simulink model "RateAdaptive_VOOmode"  (R2017b)
settings: Solver=FixedStepAuto  StartTime=0.0  StopTime=inf  FixedStep=0.001  RelTol=1e-3  EnableMultiTasking=on
undefined symbols (not defined in the file): D10, D11, D12, D2, D5, D8, D9, PTA0, PTA2, PTB9, PTC4, PTD0, PTD2, PTD3
libraries: frdmk64flib x10
settings Model: ExtModeTrigDuration=5  Creator=montema2  LastModifiedBy=puerstee
settings OptimizationCC: PassReuseOutputArgsAs=Individual arguments  MaxStackSize=64
settings DebuggingCC: ParameterTunabilityLossMsg=error
settings HardwareCC: ProdBitPerPointer=32  ProdBitPerSizeT=32  ProdBitPerPtrDiffT=32  ProdLargestAtomicInteger=Long  ProdLargestAtomicFloat=Double  ProdWordSize=32  ProdHWDeviceType=ARM Compatible->ARM Cortex
settings SFSimCC: MATLABDynamicMemAlloc=off
settings RTWCC: SystemTargetFile=ert.tlc  HardwareBoard=NXP FRDM-K64F  TemplateMakefile=ert_default_tmf  GenerateReport=on  Toolchain=GNU Tools for ARM Embedded Processors  IncludeHyperlinkInReport=on  LaunchReport=on  GenerateTraceInfo=on  GenerateTraceReport=on  GenerateTraceReportSl=on  GenerateTraceReportSf=on  GenerateTraceReportEml=on
settings CodeAppCC: ForceParamTrailComments=on  IgnoreCustomStorageClasses=off  OperatorAnnotations=on  SimulinkDataObjDesc=on  SFDataObjDesc=on  InsertBlockDesc=on
settings ERTTargetCC: SupportContinuousTime=on

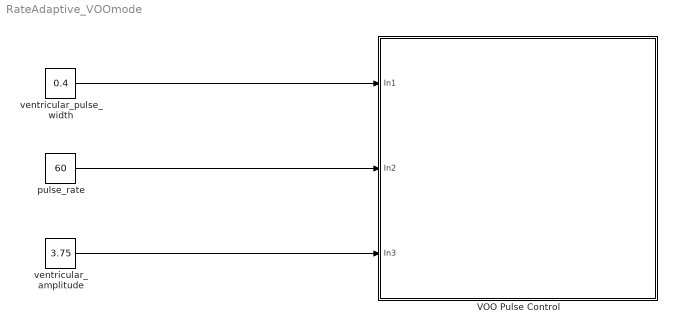
== system RateAdaptive_VOOmode ==
  VOO Pulse Control : Subsystem
  pulse_rate : Constant  Value=60  OutDataTypeStr=single
  ventricular_amplitude : Constant  Value=3.75
  ventricular_pulse_width : Constant  Value=0.4
  wires:
  ventricular_pulse_width/1 -> VOO Pulse Control/1(In1)
  pulse_rate/1 -> VOO Pulse Control/2(In2)
  ventricular_amplitude/1 -> VOO Pulse Control/3(In3)

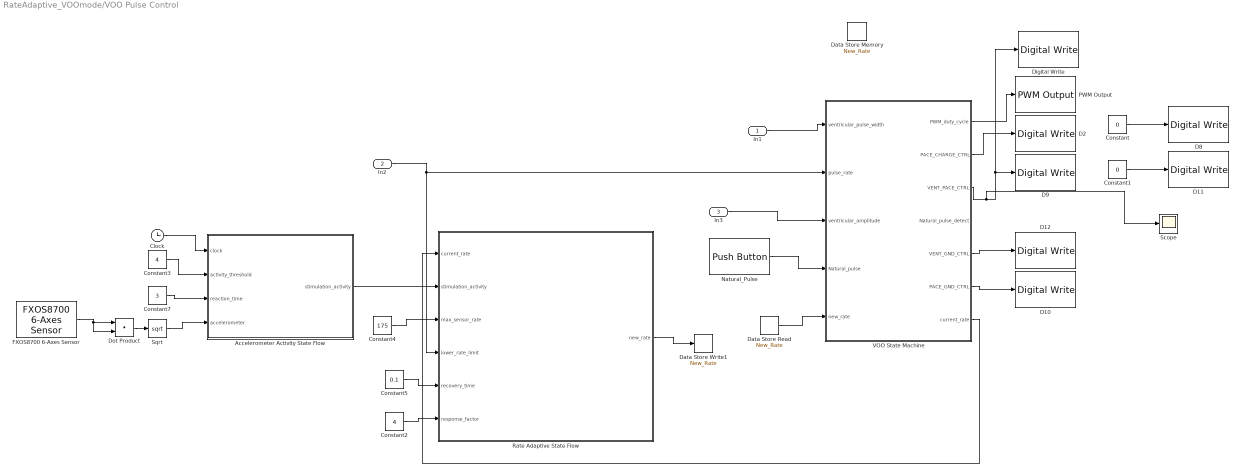
== system RateAdaptive_VOOmode/VOO Pulse Control ==
  In1 : Inport
  In2 : Inport  Port=2
  In3 : Inport  Port=3
  "Accelerometer Activity State Flow " : Stateflow chart  TreatAsAtomicUnit=on
  Clock : Clock
  Constant : Constant  Value=0
  Constant1 : Constant  Value=0
  Constant2 : Constant  Value=4  OutDataTypeStr=single
  Constant3 : Constant  Value=4  OutDataTypeStr=single
  Constant4 : Constant  Value=175  OutDataTypeStr=single
  Constant5 : Constant  Value=0.1  OutDataTypeStr=single
  Constant7 : Constant  Value=3  OutDataTypeStr=single
  D10 : frdmk64flib/Digital Write  Whichpin=PTD0 (D10)
      settings: SourceProductName=Simulink Coder Support Package for NXP FRDM-K64F Board
  D11 : frdmk64flib/Digital Write  Whichpin=PTD2 (D11)
      settings: SourceProductName=Simulink Coder Support Package for NXP FRDM-K64F Board
  D12 : frdmk64flib/Digital Write  Whichpin=PTD3 (D12)
      settings: SourceProductName=Simulink Coder Support Package for NXP FRDM-K64F Board
  D2 : frdmk64flib/Digital Write  Whichpin=PTB9 (D2)
      settings: SourceProductName=Simulink Coder Support Package for NXP FRDM-K64F Board
  D8 : frdmk64flib/Digital Write  Whichpin=PTA0 (D8)
      settings: SourceProductName=Simulink Coder Support Package for NXP FRDM-K64F Board
  D9 : frdmk64flib/Digital Write  Whichpin=PTC4 (D9)
      settings: SourceProductName=Simulink Coder Support Package for NXP FRDM-K64F Board
  Data Store Memory : DataStoreMemory  DataStoreName=New_Rate  ReadBeforeWriteMsg=warning  WriteAfterWriteMsg=warning  WriteAfterReadMsg=warning  InitialValue=60  ShowAdditionalParam=off  OutDataTypeStr=single
  Data Store Read : DataStoreRead  DataStoreName=New_Rate  DataStoreElements=New_Rate
  Data Store Write1 : DataStoreWrite  DataStoreName=New_Rate  DataStoreElements=New_Rate
  Digital Write : frdmk64flib/Digital Write  Whichpin=RED_LED
      settings: SourceProductName=Simulink Coder Support Package for NXP FRDM-K64F Board
  Dot Product : DotProduct  InputSameDT=on  OutDataTypeStr=Inherit: Inherit via internal rule
  FXOS8700 6-Axes Sensor : frdmk64flib/FXOS8700 6-Axes Sensor  Activesensor=Accelerometer only  ODR=800Hz  HybridODR=400Hz  Accelfullrange=-4g to +4g  SampleTime=-1
      settings: SourceProductName=Simulink Coder Support Package for NXP FRDM-K64F Board
  Natural_Pulse : frdmk64flib/Push Button  Whichswitch=SW2  SampleTime1=-1
      settings: SourceProductName=Simulink Coder Support Package for NXP FRDM-K64F Board
  PWM Output : frdmk64flib/PWM Output  Whichpin=PTA2 (D5)  InitialFrequency=1000  InitialDutyCycle=0
      settings: SourceProductName=Simulink Coder Support Package for NXP FRDM-K64F Board
  "Rate Adaptive State Flow " : Stateflow chart  TreatAsAtomicUnit=on
  Scope : Scope
  Sqrt : Sqrt  SaturateOnIntegerOverflow=on
  VOO State Machine : Stateflow chart  TreatAsAtomicUnit=on
  wires:
  In1/1 -> VOO State Machine/1(ventricular_pulse_width)
  VOO State Machine/1(PWM_duty_cycle) -> PWM Output/1
  VOO State Machine/3(VENT_PACE_CTRL) -> Scope/1, Digital Write/1, D9/1
  In2/1 -> "Rate Adaptive State Flow "/4(lower_rate_limit), VOO State Machine/2(pulse_rate)
  VOO State Machine/2(PACE_CHARGE_CTRL) -> D2/1
  VOO State Machine/5(VENT_GND_CTRL) -> D12/1
  VOO State Machine/6(PACE_GND_CTRL) -> D10/1
  Constant/1 -> D8/1
  Constant1/1 -> D11/1
  Natural_Pulse/1 -> VOO State Machine/4(Natural_pulse)
  In3/1 -> VOO State Machine/3(ventricular_amplitude)
  Clock/1 -> "Accelerometer Activity State Flow "/1(clock)
  Constant7/1 -> "Accelerometer Activity State Flow "/3(reaction_time)
  "Accelerometer Activity State Flow "/1(stimulation_activity) -> "Rate Adaptive State Flow "/2(stimulation_activity)
  Constant4/1 -> "Rate Adaptive State Flow "/3(max_sensor_rate)
  Constant3/1 -> "Accelerometer Activity State Flow "/2(activity_threshold)
  Constant5/1 -> "Rate Adaptive State Flow "/5(recovery_time)
  Constant2/1 -> "Rate Adaptive State Flow "/6(response_factor)
  FXOS8700 6-Axes Sensor/1 -> Dot Product/1, Dot Product/2
  Dot Product/1 -> Sqrt/1
  Sqrt/1 -> "Accelerometer Activity State Flow "/4(accelerometer)
  Data Store Read/1 -> VOO State Machine/5(new_rate)
  "Rate Adaptive State Flow "/1(new_rate) -> Data Store Write1/1
  VOO State Machine/7(current_rate) -> "Rate Adaptive State Flow "/1(current_rate)

== stateflow chart RateAdaptive_VOOmode/VOO Pulse Control/Rate Adaptive State Flow  ==
  note: Rate Adaptive State Flow
      | This state flow controls the pacing rate depending on if stimulation activity was detected in the Accelerometer Activity State Flow.
      | In order to calculate the rate of increase and rate of decrease the DCM parameters for Maximum Sensor Rate, Lower Rate Limit, Recovery Time,
      | and Response Factor are needed.
      | This state flow outputs new_rate which is an updated rate used in the Pulsing State Flow. It takes, as input, current_rate which is the most
      | recently used rate in the Pulse State Flow.
  note: Constant Lower Rate State
      | Maintains the output new_rate at the Lower Rate Limit
      | This state will only be returned to if the rate has decreased gradually
      | to the Lower Rate Limit on its own
  state const_lower_rate
    entry:new_rate = lower_rate_limit
  note: Increasing Rate State
      | If the stimulation activity becomes true and we have not
      | already reached the Maximum Sensor rate, this state is used.
      | Every second the new rate is calculated and updated if the newly
      | calculated rate will not go above the Maximum Sensor Rate
  state decreasing_rate
    entry:
    new_rate=current_rate + (lower_rate_limit - max_sensor_rate)/(60*recovery_time)
  state increasing_rate
    entry:
    new_rate=current_rate +  (max_sensor_rate/lower_rate_limit)*response_factor
  note: Decreasing Rate State
      | If the stimulation activity ever becomes false, this state
      | is used. Every second the new rate is calculated and updated
      | if the newly calculated rate will not go below the Lower Rate Limit
  state const_max_rate
    entry: new_rate=max_sensor_rate;
  note: Constant Max Rate State
      | If the rate has increased to the Maximum Sensor Rate this state is used.
      | Maintains the output new_rate at the Maximum Sensor Rate as long
      | as the stimulation activity stays true
  (default) -> const_lower_rate
  decreasing_rate -> const_lower_rate [order 2] : [after((1000),msec) && current_rate + (lower_rate_limit - max_sensor_rate)/(60*recovery_time) <= lower_rate_limit]
  const_lower_rate -> increasing_rate : [stimulation_activity==true]
  decreasing_rate -> decreasing_rate [order 3] : [after((1000),msec) && current_rate + (lower_rate_limit - max_sensor_rate)/(60*recovery_time) > lower_rate_limit]
  increasing_rate -> increasing_rate [order 3] : [(current_rate +  (max_sensor_rate/lower_rate_limit)*response_factor) < max_sensor_rate && after((1000),msec)]
  increasing_rate -> decreasing_rate [order 1] : [stimulation_activity==false]
  decreasing_rate -> increasing_rate [order 1] : [stimulation_activity==true]
  const_max_rate -> decreasing_rate : [stimulation_activity==false]
  increasing_rate -> const_max_rate [order 2] : [(current_rate +  (max_sensor_rate/lower_rate_limit)*response_factor) >= max_sensor_rate && after((1000),msec)]
  data: new_rate output single; current_rate input single; stimulation_activity input boolean; max_sensor_rate input single; lower_rate_limit input single; recovery_time input single; response_factor input single; posRoC local single; negRoC local single

== stateflow chart RateAdaptive_VOOmode/VOO Pulse Control/Accelerometer Activity State Flow  ==
  note: Accelerometer Activity State Flow
      | Takes input from the accelerometer as well as the DCM inputs for Activity Threshold and Reaction Time
      | and calculates whether the accelerometer data over one period of Reaction Time should be considered as
      | stimulation activity
  note: True State
      | True state immediatley returns to the counter state (while restarting the clock
      | and the counter) to check if stimulation activity should stay true
      | This state is entered if 2 or more samples record accelerometer activity
      | greater than the activity threshold.
  note: False State
      | Initialization state and false state sets stimulation activity
      | to false and resets the counter.
      | The only way to move out of this state is to detect
      | accelerometer activity greater than the activity threshold.
  state true_state
    entry:
    stimulation_activity = true;
    counter=0;
  state false_state
    entry:
    stimulation_activity = false;
    counter=0;
  note: Count State
      | Count state increments the counter which stores the number
      | of times acceleration activity has occured greater than activity
      | threshold within a reaction time cycle
      | This state occurs if accelerometer activity greater than the
      | activity threshold was detected, and it hasn't been a full
      | cycle of reaction time since the first activity
  note: No Count State
      | This state occurs if no accelerometer activity greater
      | than the activity threshold was detected, but it hasn't been
      | a full cycle of reaction time since the first activity (since
      | false or true state)
  state no_count_state
    entry:
    compare=clock-starttime;
  state count_state
    entry:
    counter=counter+1;
    compare=clock-starttime;
  note: No Count State and Count State sample the accelerometer data 20 times per reaction time cycle
  (default) -> false_state
  no_count_state -> false_state [order 3] : [compare>=reaction_time]
  count_state -> false_state [order 4] : [compare>=reaction_time]
  false_state -> count_state : [accelerometer >= activity_threshold]
      | {starttime=clock}
  true_state -> count_state : {starttime=clock}
  count_state -> true_state [order 1] : [counter>=2]
  no_count_state -> count_state [order 1] : [accelerometer >= activity_threshold && compare < reaction_time && after(reaction_time/20,sec)]
  count_state -> no_count_state [order 3] : [compare < reaction_time && after(reaction_time/20,sec)]
  no_count_state -> no_count_state [order 2] : [compare < reaction_time && after(reaction_time/20,sec)]
  count_state -> count_state [order 2] : [accelerometer >= activity_threshold && compare < reaction_time && after(reaction_time/20,sec)]
  data: clock input; stimulation_activity output boolean; activity_threshold input single; reaction_time input single; accelerometer input double; compare local; counter local int16; starttime local

== stateflow chart RateAdaptive_VOOmode/VOO Pulse Control/VOO State Machine ==
  note: Switch States:
      | true=closed
      | false=open
  state start_state
    entry:VENT_PACE_CTRL=false;
    VENT_GND_CTRL=true;
    PACE_CHARGE_CTRL=true;
    PACE_GND_CTRL=true;
    PWM_duty_cycle=((ventricular_amplitude)*20);
    current_rate = pulse_rate;
  state current_into_heart
    entry:
    PACE_CHARGE_CTRL=false;
    VENT_GND_CTRL=false;
    VENT_PACE_CTRL=true;
    current_rate=new_rate;
  state current_out_of_heart
    entry:
    VENT_PACE_CTRL=false;
    PACE_CHARGE_CTRL=true;
    VENT_GND_CTRL=true;
    current_rate=new_rate;
  state natural_pace
    entry: Natural_pulse_detect=true;
    exit: Natural_pulse_detect=false;
  (default) -> start_state
  start_state -> current_into_heart [order 1] : [after((60000/current_rate),msec)]
  current_into_heart -> natural_pace [order 2] : [Natural_pulse==true]
  start_state -> natural_pace [order 2] : [Natural_pulse==true]
  natural_pace -> start_state : [Natural_pulse==false]
  current_into_heart -> current_out_of_heart [order 1] : [after((ventricular_pulse_width),msec)]
  current_out_of_heart -> current_into_heart [order 1] : [after((60000/current_rate)-(ventricular_pulse_width),msec)]
  current_out_of_heart -> natural_pace [order 2] : [Natural_pulse==true]
  data: ventricular_pulse_width input double; pulse_rate input single; ventricular_amplitude input double; PWM_duty_cycle output double [0..100]; PACE_CHARGE_CTRL output boolean; VENT_PACE_CTRL output boolean; Natural_pulse_detect output; VENT_GND_CTRL output boolean; PACE_GND_CTRL output boolean; Natural_pulse input boolean; new_rate input single; current_rate output single
